simulink model "VTOL_sim"  (R2015a)
settings: Solver=ode45  StartTime=0.0  StopTime=200  RelTol=1e-3
InitFcn:
  | param
undefined symbols (not defined in the file or in its folder): drawVTOL, P, VTOL_ctrl
settings Model: Creator=beard  LastModifiedBy=beard
settings DataIOCC: SignalLoggingSaveFormat=ModelDataLogs
settings OptimizationCC: ExpressionDepthLimit=2147483647  InitFltsAndDblsToZero=on
settings DebuggingCC: UnderspecifiedInitializationDetection=Classic  MergeDetectMultiDrivingBlocksExec=none  SolverPrmCheckMsg=warning  FcnCallInpInsideContextMsg=UseLocalSettings  StateNameClashWarn=warning
settings GRTTargetCC: CombineOutputUpdateFcns=off  GRTInterface=on

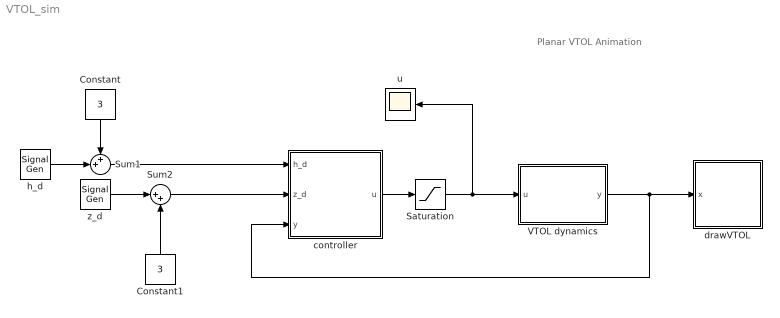
== system VTOL_sim ==
  note: Planar VTOL Animation
  Constant : Constant  Value=3
  Constant1 : Constant  Value=3
  Saturation : Saturate  UpperLimit=P.fmax  LowerLimit=0
  Sum1 : Sum  Inputs=++|
  Sum2 : Sum  Inputs=|++
  VTOL dynamics : Subsystem
  controller : Subsystem
  drawVTOL : Subsystem
      mask Display: image(imread('tv.jpg'))
  h_d : SignalGenerator  WaveForm=square  Amplitude=2.5  Frequency=.02
  u : Scope
      settings: TimeRange=200  YMin=0  YMax=10  SaveName=ScopeData2
  z_d : SignalGenerator  WaveForm=square  Amplitude=2.5  Frequency=.015
  wires:
  Constant/1 -> Sum1/1
  h_d/1 -> Sum1/2
  Sum2/1 -> controller/2(z_d)
  z_d/1 -> Sum2/1
  Constant1/1 -> Sum2/2
  Saturation/1 -> VTOL dynamics/1(u), u/1
  controller/1(u) -> Saturation/1
  Sum1/1 -> controller/1(h_d)
  VTOL dynamics/1(y) -> controller/3(y), drawVTOL/1(x)

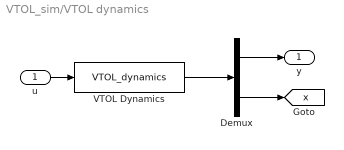
== system VTOL_sim/VTOL dynamics ==
  u : Inport
  Demux : Demux  Outputs=[3;6]
  VTOL Dynamics : S-Function  FunctionName=VTOL_dynamics  Parameters=AP
  y : Outport
  tag scope: x=global
  wires:
  u/1 -> VTOL Dynamics/1
  Demux/1 -> y/1
  VTOL Dynamics/1 -> Demux/1
  Demux/2 -> [x]

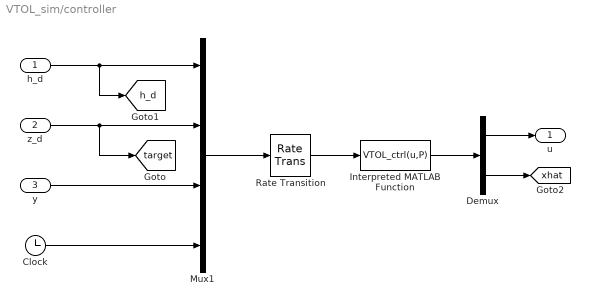
== system VTOL_sim/controller ==
  h_d : Inport
  z_d : Inport  Port=2
  y : Inport  Port=3
  Clock : Clock
  Demux : Demux  Outputs=[2;6]
  Interpreted MATLAB Function : MATLABFcn  MATLABFcn=VTOL_ctrl(u,P)  OutputDimensions=2+6
  Mux1 : Mux
  Rate Transition : RateTransition  OutPortSampleTime=P.Ts
  u : Outport
  tag scope: h_d=global, target=global, xhat=global
  wires:
  Mux1/1 -> Rate Transition/1
  h_d/1 -> [h_d], Mux1/1
  Clock/1 -> Mux1/4
  Rate Transition/1 -> Interpreted MATLAB Function/1
  y/1 -> Mux1/3
  z_d/1 -> [target], Mux1/2
  Interpreted MATLAB Function/1 -> Demux/1
  Demux/1 -> u/1
  Demux/2 -> [xhat]

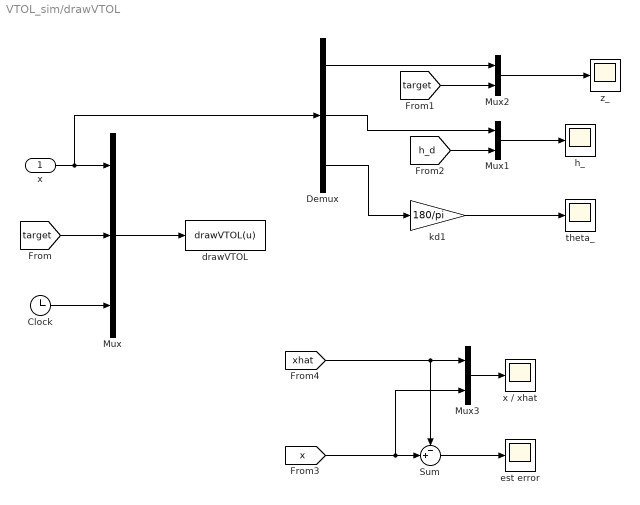
== system VTOL_sim/drawVTOL ==
  x : Inport
  Clock : Clock
  Demux : Demux  Outputs=3
  Mux : Mux  Inputs=3
  Mux1 : Mux  Inputs=2
  Mux2 : Mux  Inputs=2
  Mux3 : Mux  Inputs=2
  Sum : Sum  Inputs=-+|
  drawVTOL : MATLABFcn  MATLABFcn=drawVTOL(u)  OutputDimensions=0  SampleTime=0.1
  est error : Scope
      settings: TimeRange=40  YMin=-6  YMax=7
  h_ : Scope
      settings: TimeRange=200  YMin=0  YMax=6  SaveName=ScopeData3
  kd1 : Gain  Gain=180/pi
  theta_ : Scope
      settings: TimeRange=200  YMin=-60  YMax=60  SaveName=ScopeData5
  x / xhat : Scope
      settings: TimeRange=40  YMin=-3.5  YMax=6
  z_ : Scope
      settings: TimeRange=200  YMin=0  YMax=6  SaveName=ScopeData4
  wires:
  Mux/1 -> drawVTOL/1
  x/1 -> Demux/1, Mux/1
  Clock/1 -> Mux/3
  [target] -> Mux/2
  Mux1/1 -> h_/1
  Mux2/1 -> z_/1
  kd1/1 -> theta_/1
  Demux/3 -> kd1/1
  Demux/1 -> Mux2/1
  [target] -> Mux2/2
  Demux/2 -> Mux1/1
  [h_d] -> Mux1/2
  Mux3/1 -> x / xhat/1
  Sum/1 -> est error/1
  [xhat] -> Mux3/1, Sum/1
  [x] -> Mux3/2, Sum/2
